simulink library "saturateRudderAngle"  (R2018a)
settings: Solver=VariableStepAuto  StartTime=0.0  StopTime=10.0  RelTol=1e-3
undefined symbols (not defined in the file): plant
libraries: simulink x1
settings Model: Creator=mitch  LastModifiedBy=mitch

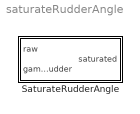
== system saturateRudderAngle ==
  "SaturateRudderAngle " : Subsystem

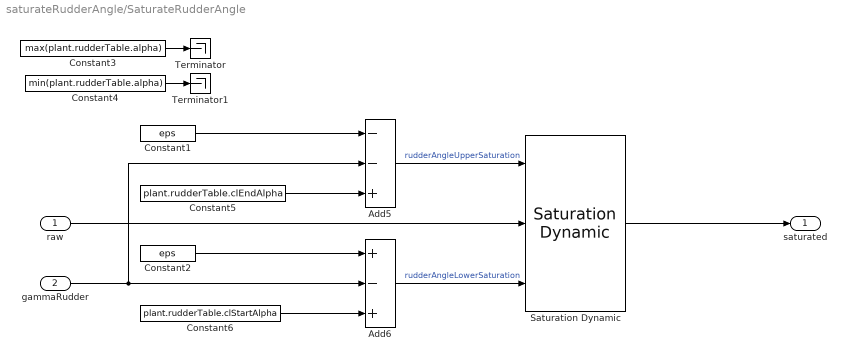
== system saturateRudderAngle/SaturateRudderAngle  ==
  raw : Inport
  gammaRudder : Inport  Port=2
  Add5 : Sum  Inputs=--+
  Add6 : Sum  Inputs=+-+
  Constant1 : Constant  Value=eps
  Constant2 : Constant  Value=eps
  Constant3 : Constant  Value=max(plant.rudderTable.alpha)
  Constant4 : Constant  Value=min(plant.rudderTable.alpha)
  Constant5 : Constant  Value=plant.rudderTable.clEndAlpha
  Constant6 : Constant  Value=plant.rudderTable.clStartAlpha
  Saturation Dynamic : simulink/Discontinuities/Saturation Dynamic  OutMin=[]  OutMax=[]  OutDataTypeStr=Inherit: Same as second input  OutDataType=fixdt(1, 16)  OutScaling=2^-10  DoSatur=off
  Terminator : Terminator
  Terminator1 : Terminator
  saturated : Outport
  wires:
  Add5/1 -> Saturation Dynamic/1  "rudderAngleUpperSaturation"
  Add6/1 -> Saturation Dynamic/3  "rudderAngleLowerSaturation"
  gammaRudder/1 -> Add5/2, Add6/2
  Constant6/1 -> Add6/3
  Constant2/1 -> Add6/1
  raw/1 -> Saturation Dynamic/2
  Constant1/1 -> Add5/1
  Saturation Dynamic/1 -> saturated/1
  Constant3/1 -> Terminator/1
  Constant4/1 -> Terminator1/1
  Constant5/1 -> Add5/3
